simulink model "LAB2_Part2"  (R2023a)
settings: Solver=FixedStepDiscrete  StartTime=0.0  StopTime=inf  FixedStep=0.01  RelTol=1e-3  EnableMultiTasking=on
values from neighbouring files (symbols this model uses):
  ccw_dir = 0    [Stepper_Motor_Script.m]
  cw_dir = 0    [Stepper_Motor_Script.m]
  drive_mode = 1    [Stepper_Motor_Script.m]
  freq = 1    [Stepper_Motor_Script.m]
  hold_pos = 0    [Stepper_Motor_Script.m]
  motor_enable = 0    [Stepper_Motor_Script.m]
undefined symbols (not defined in the file or in its folder): LF
libraries: instrumentseriallib x5, simulink x2, hdlsllib x1
settings Model: Creator=User  LastModifiedBy=AbsoluteZeno
settings SolverCC: AllowMultiTaskInputOutput=on  ConcurrentTasks=on  AutoInsertRateTranBlk=on

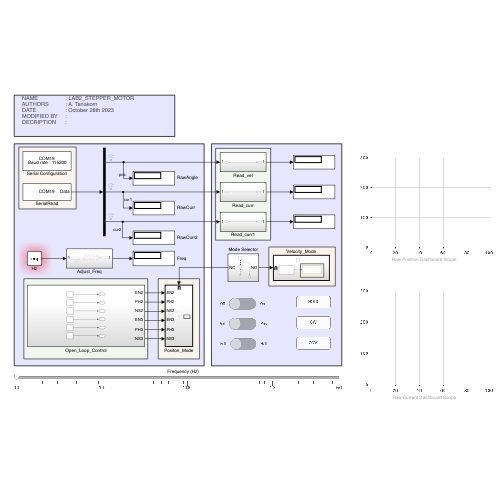
[thumbnail: Simulink's stored preview of the top-level diagram]
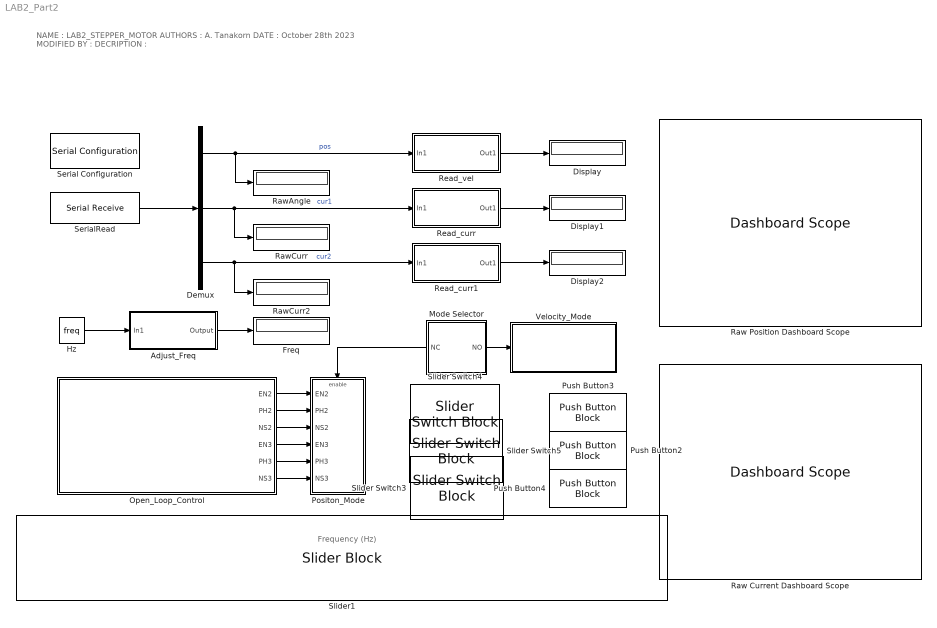
== system LAB2_Part2 ==
  note: NAME                  : LAB2_STEPPER_MOTOR
      |     AUTHORS           : A. Tanakorn
      |     DATE                   : October 28th 2023
      |     MODIFIED BY     :
      |     DECRIPTION      :
  note: Frequency (Hz)
  Adjust_Freq : Subsystem
  Demux : Demux  Outputs=3
  Display : Display
  Display1 : Display
  Display2 : Display
  Freq : Display
  Hz : Constant  Value=freq  OutDataTypeStr=double
  Mode Selector : Subsystem
      settings: PortSchema="{\"entries\":[{\"content\":{\"sides\":[{\"content\":{},\"type\":\"ConnectorPlacement.EquallySpacedRectSide\",\"uuid\":\"9fa117e9-068f-4873-871c-793b702c6091\"},{\"content\":{\"side\":\"RIGHT\"},\"type\":\"ConnectorPlacement.EquallySpacedRectSide\",\"uuid\":\"19297395-6cd8-433d-a702-744f2e67145d\"},{\"content\":{\"connectorIds\":[\"Out2\"],\"side\":\"TOP\"},\"type\":\"ConnectorPlacement.EquallySpacedRectSide\",\"uuid\":\"1c0d5175-0616-4474-94e1-5874b3e5fd11\"},{\"content\":{\"connectorIds\":[\"Out1\"],\"side\":\"BOTTOM\"},\"type\":\"ConnectorPlacement.EquallySpacedRectSide\",\"uuid\":\"c07c49ab-d11a-4a00-a3f8-fceddddb600a\"}]},\"type\":\"ConnectorPlacement.EquallySpacedConnector\",\"uuid\":\"dc9f3a1e-f7ef-41e6-9ea6-55363284eb30\"}],\"packageUris\":[\"http://schema.mathworks.com/mf0/Connector/R2020b\"],\"version\":\"1.0\"}"
  Open_Loop_Control : Subsystem
  Positon_Mode : Subsystem  TreatAsAtomicUnit=on
  Push Button2 : PushButtonBlock  ButtonText=CW  OffValue=0.000000
  Push Button3 : PushButtonBlock  ButtonText=HOLD  OffValue=0.000000
  Push Button4 : PushButtonBlock  ButtonText=CCW  OffValue=0.000000
  Raw Current Dashboard Scope : DashboardScope  Ymin=0  Ymax=300  UpdateMode=Scroll
  Raw Position Dashboard Scope : DashboardScope  Ymin=0  Ymax=300  UpdateMode=Scroll
  RawAngle : Display
  RawCurr : Display
  RawCurr2 : Display
  Read_curr : Subsystem
  Read_curr1 : Subsystem
  Read_vel : Subsystem
  Serial Configuration : instrumentseriallib/Serial Configuration  Priority=-200000  PortSel=COM19  Port=COM19  ComPort=COM19  BaudRate=115200  DataBits=8  Parity=none  StopBits=1  ByteOrder=little-endian  FlowControl=none  Timeout=10  SimulateUsing=Interpreted execution  BlockInModel=on  aMode=1
      settings: LibrarySourceBlock=c2000lib/Host Communication/Serial Configuration
  SerialRead : instrumentseriallib/Serial Receive  Priority=1  PortSel=COM19  Port=COM19  ComPort=COM19  DataType=uint16  SaveDataType=uint8  ToggleHeader=on  Header=[69]  ToggleTerminator=on  Terminator=LF ('\n')  CustomTerminator=[]  InputFormat=Column major  ToggleDataSize=on  DataSize=[3]  EnableBlockingMode=on  ActionDataUnavailable=Output last received value  ActionWhenDataUnavailable=Output last received value  CustomValue=0  SampleTime=-1  SimulateUsing=Interpreted execution  BlockInModel=on  aMode=1
  Slider Switch3 : SliderSwitchBlock  LabelPosition=Hide
      settings: Values={{'Full', 'Half'}, [1 2]}
  Slider Switch4 : SliderSwitchBlock  LabelPosition=Hide
      settings: Values={{'Off', 'On'}, [0 1]}
  Slider Switch5 : SliderSwitchBlock  LabelPosition=Hide
      settings: Values={{'Vel', 'Pos'}, [1 0]}
  Slider1 : SliderBlock  LabelPosition=Hide  ScaleMin=1  ScaleMax=6000  ScaleType=Log
  Velocity_Mode : Subsystem  TreatAsAtomicUnit=on
  wires:
  Read_curr/1(Out1) -> Display1/1
  Demux/1 -> RawAngle/1, Read_vel/1(In1)  "pos"
  Read_vel/1(Out1) -> Display/1
  Hz/1 -> Adjust_Freq/1(In1)
  SerialRead/1 -> Demux/1
  Demux/2 -> RawCurr/1, Read_curr/1(In1)  "cur1"
  Adjust_Freq/1(Output) -> Freq/1
  Demux/3 -> RawCurr2/1, Read_curr1/1(In1)  "cur2"
  Read_curr1/1(Out1) -> Display2/1
  Mode Selector/2(NC) -> Positon_Mode/Enable
  Mode Selector/1(NO) -> Velocity_Mode/Enable
  Open_Loop_Control/1(EN2) -> Positon_Mode/1(EN2)
  Open_Loop_Control/2(PH2) -> Positon_Mode/2(PH2)
  Open_Loop_Control/3(NS2) -> Positon_Mode/3("NS2 ")
  Open_Loop_Control/4(EN3) -> Positon_Mode/4(EN3)
  Open_Loop_Control/5(PH3) -> Positon_Mode/5(PH3)
  Open_Loop_Control/6(NS3) -> Positon_Mode/6(NS3)

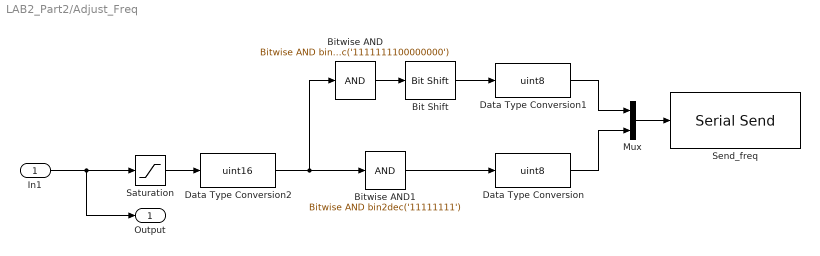
== system LAB2_Part2/Adjust_Freq ==
  In1 : Inport
  Bit Shift : hdlsllib/Logic and Bit Operations/Bit Shift  mode=Shift Right Logical  N=8
  Bitwise AND : simulink/Logic and Bit Operations/Bitwise Operator  logicop=AND  UseBitMask=on  BitMask=bin2dec('1111111100000000')  BitMaskRealWorld=Stored Integer
  Bitwise AND1 : simulink/Logic and Bit Operations/Bitwise Operator  logicop=AND  UseBitMask=on  BitMask=bin2dec('11111111')  BitMaskRealWorld=Stored Integer
  Data Type Conversion : DataTypeConversion  OutDataTypeStr=uint8  SaturateOnIntegerOverflow=off  RndMeth=Floor
  Data Type Conversion1 : DataTypeConversion  OutDataTypeStr=uint8  SaturateOnIntegerOverflow=off  RndMeth=Floor
  Data Type Conversion2 : DataTypeConversion  OutDataTypeStr=uint16  SaturateOnIntegerOverflow=off  RndMeth=Floor
  Mux : Mux  Inputs=2
  Saturation : Saturate  UpperLimit=20000  LowerLimit=5
  Send_freq : instrumentseriallib/Serial Send  Priority=1  PortSel=COM19  Port=COM19  ComPort=COM19  Header=[69]  Terminator=<none>  CustomTerminator=[123]  EnableBlockingMode=on  SimulateUsing=Interpreted execution  BlockInModel=on  aMode=1
  Output : Outport
  wires:
  Mux/1 -> Send_freq/1
  Saturation/1 -> Data Type Conversion2/1
  Data Type Conversion/1 -> Mux/2
  Bitwise AND/1 -> Bit Shift/1
  Bitwise AND1/1 -> Data Type Conversion/1
  Data Type Conversion2/1 -> Bitwise AND1/1, Bitwise AND/1
  Data Type Conversion1/1 -> Mux/1
  Bit Shift/1 -> Data Type Conversion1/1
  In1/1 -> Output/1, Saturation/1

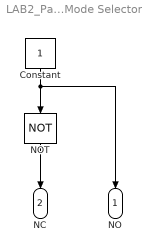
== system LAB2_Part2/Mode Selector ==
  Constant : Constant
  NOT : Logic  Operator=NOT  IconShape=distinctive  AllPortsSameDT=off  OutDataTypeStr=boolean
  NO : Outport
  NC : Outport  Port=2
  wires:
  NOT/1 -> NC/1
  Constant/1 -> NO/1, NOT/1

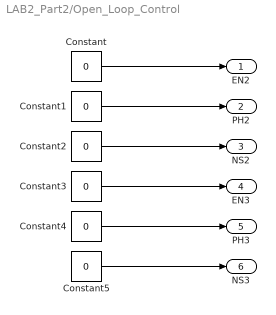
== system LAB2_Part2/Open_Loop_Control ==
  Constant{,1..5} (6 alike) : Constant  Value=0
  EN2 : Outport
  PH2 : Outport  Port=2
  NS2 : Outport  Port=3
  EN3 : Outport  Port=4
  PH3 : Outport  Port=5
  NS3 : Outport  Port=6
  wires:
  Constant/1 -> EN2/1
  Constant1/1 -> PH2/1
  Constant2/1 -> NS2/1
  Constant3/1 -> EN3/1
  Constant4/1 -> PH3/1
  Constant5/1 -> NS3/1

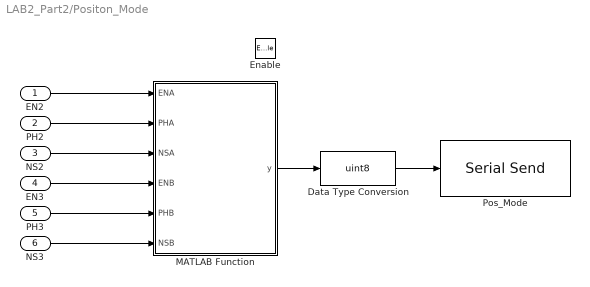
== system LAB2_Part2/Positon_Mode ==
  EN2 : Inport
  PH2 : Inport  Port=2
  "NS2 " : Inport  Port=3
  EN3 : Inport  Port=4
  PH3 : Inport  Port=5
  NS3 : Inport  Port=6
  Enable : EnablePort  StatesWhenEnabling=reset
  Data Type Conversion : DataTypeConversion  OutDataTypeStr=uint8  SaturateOnIntegerOverflow=off  RndMeth=Floor
  MATLAB Function : MATLAB Function  TreatAsAtomicUnit=on
  Pos_Mode : instrumentseriallib/Serial Send  Priority=1  PortSel=COM19  Port=COM19  ComPort=COM19  Header=[71]  Terminator=LF ('\n')  CustomTerminator=[123]  EnableBlockingMode=on  SimulateUsing=Interpreted execution  BlockInModel=on  aMode=1
  wires:
  MATLAB Function/1(y) -> Data Type Conversion/1
  EN2/1 -> MATLAB Function/1(ENA)
  PH2/1 -> MATLAB Function/2(PHA)
  "NS2 "/1 -> MATLAB Function/3(NSA)
  EN3/1 -> MATLAB Function/4(ENB)
  PH3/1 -> MATLAB Function/5(PHB)
  NS3/1 -> MATLAB Function/6(NSB)
  Data Type Conversion/1 -> Pos_Mode/1

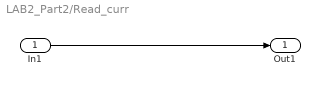
== system LAB2_Part2/Read_curr ==
  In1 : Inport
  Out1 : Outport
  wires:
  In1/1 -> Out1/1

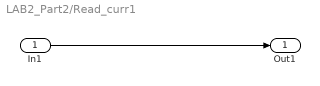
== system LAB2_Part2/Read_curr1 ==
  In1 : Inport
  Out1 : Outport
  wires:
  In1/1 -> Out1/1

== system LAB2_Part2/Read_vel ==
  In1 : Inport
  Out1 : Outport
  wires:
  In1/1 -> Out1/1

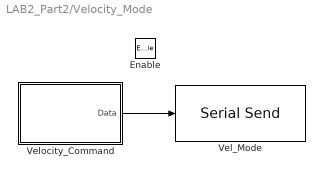
== system LAB2_Part2/Velocity_Mode ==
  Enable : EnablePort  StatesWhenEnabling=reset
  Vel_Mode : instrumentseriallib/Serial Send  Priority=1  PortSel=COM19  Port=COM19  ComPort=COM19  Header=[70]  Terminator=LF ('\n')  CustomTerminator=[123]  EnableBlockingMode=on  SimulateUsing=Interpreted execution  BlockInModel=on  aMode=1
  Velocity_Command : Subsystem
  wires:
  Velocity_Command/1(Data) -> Vel_Mode/1

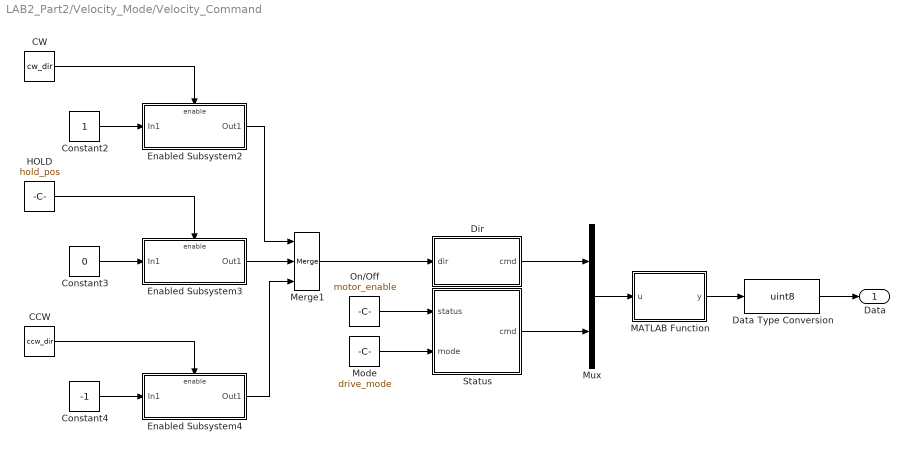
== system LAB2_Part2/Velocity_Mode/Velocity_Command ==
  CCW : Constant  Value=ccw_dir
  CW : Constant  Value=cw_dir
  Constant2 : Constant
  Constant3 : Constant  Value=0
  Constant4 : Constant  Value=-1
  Data Type Conversion : DataTypeConversion  OutDataTypeStr=uint8  SaturateOnIntegerOverflow=off  RndMeth=Floor
  Dir : MATLAB Function  TreatAsAtomicUnit=on
  Enabled Subsystem2 : Subsystem  TreatAsAtomicUnit=on
  Enabled Subsystem3 : Subsystem  TreatAsAtomicUnit=on
  Enabled Subsystem4 : Subsystem  TreatAsAtomicUnit=on
  HOLD : Constant  Value=hold_pos
  MATLAB Function : MATLAB Function  TreatAsAtomicUnit=on
  Merge1 : Merge  Inputs=3
  Mode : Constant  Value=drive_mode
  Mux : Mux  Inputs=2
  On/Off : Constant  Value=motor_enable
  Status : MATLAB Function  TreatAsAtomicUnit=on
  Data : Outport
  wires:
  Enabled Subsystem3/1(Out1) -> Merge1/2
  HOLD/1 -> Enabled Subsystem3/Enable
  Merge1/1 -> Dir/1(dir)
  Dir/1(cmd) -> Mux/1
  Mode/1 -> Status/2(mode)
  On/Off/1 -> Status/1(status)
  CCW/1 -> Enabled Subsystem4/Enable
  Status/1(cmd) -> Mux/2
  Constant3/1 -> Enabled Subsystem3/1(In1)
  Constant4/1 -> Enabled Subsystem4/1(In1)
  Constant2/1 -> Enabled Subsystem2/1(In1)
  Enabled Subsystem2/1(Out1) -> Merge1/1
  Enabled Subsystem4/1(Out1) -> Merge1/3
  CW/1 -> Enabled Subsystem2/Enable
  Mux/1 -> MATLAB Function/1(u)
  MATLAB Function/1(y) -> Data Type Conversion/1
  Data Type Conversion/1 -> Data/1

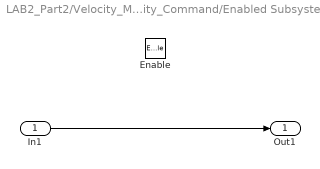
== system LAB2_Part2/Velocity_Mode/Velocity_Command/Enabled Subsystem2 ==
  In1 : Inport
  Enable : EnablePort
  Out1 : Outport
  wires:
  In1/1 -> Out1/1

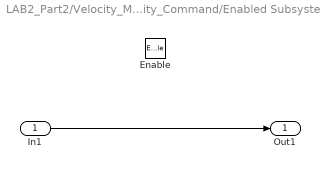
== system LAB2_Part2/Velocity_Mode/Velocity_Command/Enabled Subsystem3 ==
  In1 : Inport
  Enable : EnablePort
  Out1 : Outport
  wires:
  In1/1 -> Out1/1

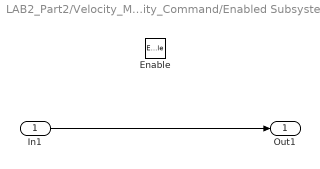
== system LAB2_Part2/Velocity_Mode/Velocity_Command/Enabled Subsystem4 ==
  In1 : Inport
  Enable : EnablePort
  Out1 : Outport
  wires:
  In1/1 -> Out1/1

== matlab function LAB2_Part2/Velocity_Mode/Velocity_Command/MATLAB Function ==
  data: u input; y output
function y = fcn(u)

y = (u(1) * 8) + (u(2) * 4) + (u(3) * 2) + u(4);

== matlab function LAB2_Part2/Positon_Mode/MATLAB Function ==
  data: ENA input; y output; PHA input; NSA input; ENB input; PHB input; NSB input
function y = fcn(ENA,PHA,NSA,ENB,PHB,NSB)
y = (ENA * 32) + (PHA * 16) + (NSA * 8) + (ENB * 4) + (PHB * 2) + (NSB);

== matlab function LAB2_Part2/Velocity_Mode/Velocity_Command/Dir ==
  data: dir input; cmd output
function cmd = fcn(dir)
    if dir == 0
        cmd = [0 0];
    elseif dir == 1
        cmd = [0 1];
    elseif dir == -1
        cmd = [1 0];
    else
        cmd = [NaN NaN];
    end
end

== matlab function LAB2_Part2/Velocity_Mode/Velocity_Command/Status ==
  data: status input; mode input; cmd output
function cmd = fcn(status,mode)
    if status == 1
        if mode == 1
            cmd = [0 1];
        elseif mode == 2
            cmd = [1 0];
        else
            cmd = [NaN NaN];
        end
    else
        cmd = [0 0];
    end
end
